simulink model "fuzzyproyecto"  (R2018a)
settings: Solver=VariableStepAuto  StartTime=0.0  StopTime=10  RelTol=1e-3
libraries: fuzblock x1
settings Model: Creator=Alvaro  LastModifiedBy=Alvaro

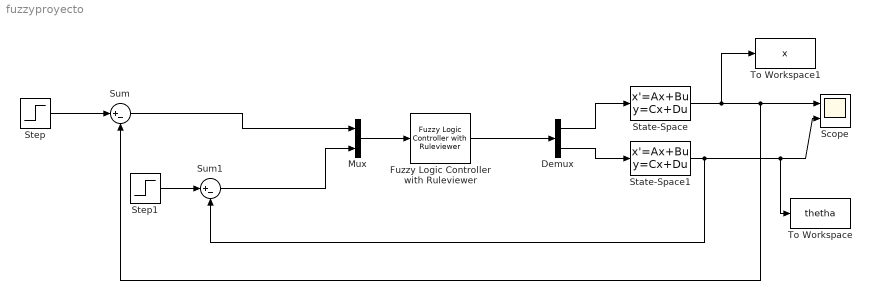
== system fuzzyproyecto ==
  Demux : Demux  Outputs=2
  Fuzzy Logic Controller with Ruleviewer : fuzblock/Fuzzy Logic  Controller  with Ruleviewer  fismatrix=robot  Ts=1
  Mux : Mux  Inputs=2
  Scope : Scope  NumInputPorts=2
  State-Space : StateSpace  A=[0 1 0 0;-4.0295 0 0 0;0 0 0 1;57.2671 0 0 0]  B=[0;39.0316;0;-207.487]  C=[0 0 1 0]  D=[0]  InitialCondition=[0.01 0 0.01 0]
  State-Space1 : StateSpace  A=[0 1 0 0;-4.0295 0 0 0;0 0 0 1;57.2671 0 0 0]  B=[0;39.0316;0;-207.487]  C=[1 0 0 0]  D=[0]  InitialCondition=[0.1 0 0.1 0]
  Step : Step  Before=0.2  After=0  SampleTime=0
  Step1 : Step  Before=0.2  After=0  SampleTime=0
  Sum : Sum  Inputs=|+-
  Sum1 : Sum  Inputs=|+-
  To Workspace : ToWorkspace  VariableName=thetha  SampleTime=-1
  To Workspace1 : ToWorkspace  VariableName=x  SampleTime=-1
  wires:
  Step/1 -> Sum/1
  Step1/1 -> Sum1/1
  Demux/1 -> State-Space/1
  Demux/2 -> State-Space1/1
  State-Space1/1 -> Sum1/2, To Workspace/1, Scope/2
  State-Space/1 -> To Workspace1/1, Scope/1, Sum/2
  Fuzzy Logic Controller with Ruleviewer/1 -> Demux/1
  Mux/1 -> Fuzzy Logic Controller with Ruleviewer/1
  Sum/1 -> Mux/1
  Sum1/1 -> Mux/2
